simulink model "e4_3"  (R2018a)
settings: Solver=FixedStepAuto  StartTime=0.0  StopTime=100.0  FixedStep=0.00001  RelTol=1e-3
settings Model: Creator=hp  LastModifiedBy=hp

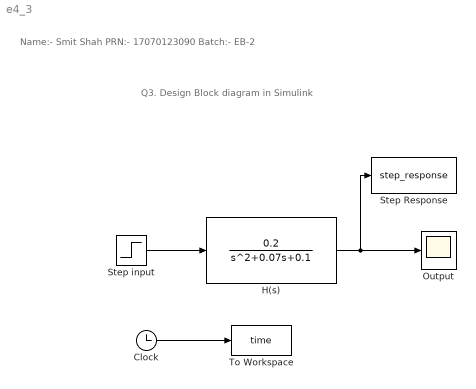
== system e4_3 ==
  note: Name:- Smit Shah PRN:- 17070123090 Batch:- EB-2
  note: Q3. Design Block diagram in Simulink
  Clock : Clock
      settings: Decimation=100
  H(s) : TransferFcn  Numerator=[0.2]  Denominator=[1 0.07 0.1]
  Output : Scope
  Step Response : ToWorkspace  VariableName=step_response  SampleTime=-1
  Step input : Step  Time=0  SampleTime=0
  To Workspace : ToWorkspace  VariableName=time  SampleTime=-1
  wires:
  Step input/1 -> H(s)/1
  H(s)/1 -> Step Response/1, Output/1
  Clock/1 -> To Workspace/1
